simulink model "AFS_DD"  (R2016b)
settings: configuration reference "CodeGenConfigSet" (kept outside this file)
values from neighbouring files (symbols this model uses):
  AFS_facLPFiltPT1_C = Calibration.Parameter    [init_AFS_DD.m]    (also in init_AFS_DD_SIL.m = Simulink.Parameter)
  AFS_tiRawSRCHi_C = Calibration.Parameter    [init_AFS_DD.m]    (also in init_AFS_DD_SIL.m = Simulink.Parameter)
  AFS_tiRawSRCLo_C = Calibration.Parameter    [init_AFS_DD.m]    (also in init_AFS_DD_SIL.m = Simulink.Parameter)
  AFS_tiRawSRCMaxDebDef_C = Calibration.Parameter    [init_AFS_DD.m]    (also in init_AFS_DD_SIL.m = Simulink.Parameter)
  AFS_tiRawSRCMaxDebOk_C = Calibration.Parameter    [init_AFS_DD.m]    (also in init_AFS_DD_SIL.m = Simulink.Parameter)
  AFS_tiRawSRCMinDebDef_C = Calibration.Parameter    [init_AFS_DD.m]    (also in init_AFS_DD_SIL.m = Simulink.Parameter)
  AFS_tiRawSRCMinDebOk_C = Calibration.Parameter    [init_AFS_DD.m]    (also in init_AFS_DD_SIL.m = Simulink.Parameter)
undefined symbols (not defined in the file or in its folder): AFS_DD_DT, Switch_conv
libraries: CXLib x7
settings Model: Creator=Colin  LastModifiedBy=Colin
settings ConfigSetRef: SourceLocation=Base Workspace

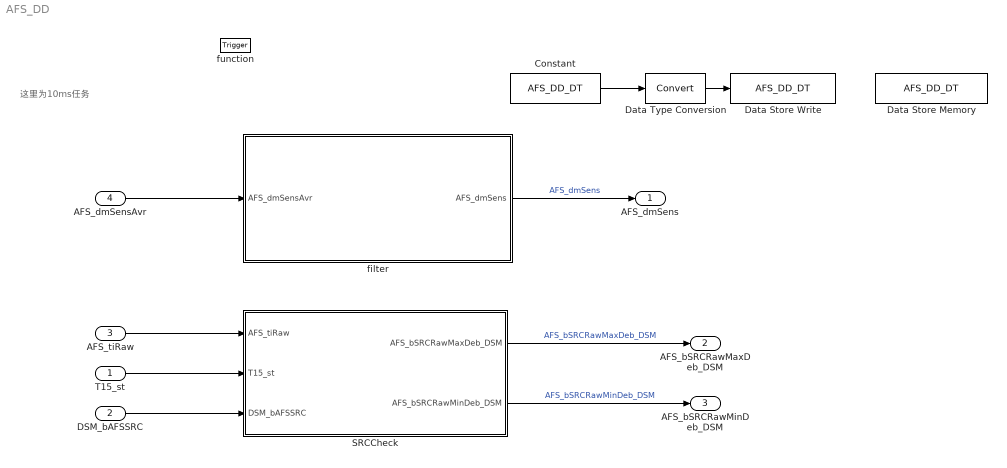
== system AFS_DD ==
  note: 这里为10ms任务
  T15_st : Inport  Description=Terminal 15 status after debouncing  OutDataTypeStr=Enum: Switch_conv
  DSM_bAFSSRC : Inport  Description=Function identifier for inhibition of the signal range check  Port=2  OutMin=0  OutMax=1  OutDataTypeStr=boolean
  AFS_tiRaw : Inport  Tag=us  Description=Raw air mass period  Port=3  OutMin=0  OutMax=107374182  OutDataTypeStr=Time_PwmHigh_us
  AFS_dmSensAvr : Inport  Tag=kg/h  Description=Averaged Sensed air mass flow  Port=4  OutMin=-8192  OutMax=8191  OutDataTypeStr=AirMassPerTime
  function : TriggerPort  TriggerType=function-call  VariantControl=Variant
  Constant : Constant  Value=AFS_DD_DT
  Data Store Memory : DataStoreMemory  DataStoreName=AFS_DD_DT  ReadBeforeWriteMsg=warning  WriteAfterWriteMsg=warning  WriteAfterReadMsg=warning  ShowAdditionalParam=off
  Data Store Write : DataStoreWrite  DataStoreName=AFS_DD_DT
  Data Type Conversion : DataTypeConversion
  SRCCheck : Subsystem
  filter : Subsystem
  AFS_dmSens : Outport  Tag=kg/h  Description=Processed air mass flow signal of the HFM sensor  OutMin=-8192  OutMax=8191  OutDataTypeStr=AirMassPerTime
  AFS_bSRCRawMaxDeb_DSM : Outport  Description=Signal range check high of the air mass flow sensor  Port=2  OutMin=0  OutMax=1  OutDataTypeStr=boolean
  AFS_bSRCRawMinDeb_DSM : Outport  Description=Signal range check low of the air mass flow sensor  Port=3  OutMin=0  OutMax=1  OutDataTypeStr=boolean
  wires:
  T15_st/1 -> SRCCheck/2(T15_st)
  DSM_bAFSSRC/1 -> SRCCheck/3(DSM_bAFSSRC)
  SRCCheck/1(AFS_bSRCRawMaxDeb_DSM) -> AFS_bSRCRawMaxDeb_DSM/1  "AFS_bSRCRawMaxDeb_DSM"
  SRCCheck/2(AFS_bSRCRawMinDeb_DSM) -> AFS_bSRCRawMinDeb_DSM/1  "AFS_bSRCRawMinDeb_DSM"
  Constant/1 -> Data Type Conversion/1
  AFS_tiRaw/1 -> SRCCheck/1(AFS_tiRaw)
  AFS_dmSensAvr/1 -> filter/1(AFS_dmSensAvr)
  filter/1(AFS_dmSens) -> AFS_dmSens/1  "AFS_dmSens"
  Data Type Conversion/1 -> Data Store Write/1

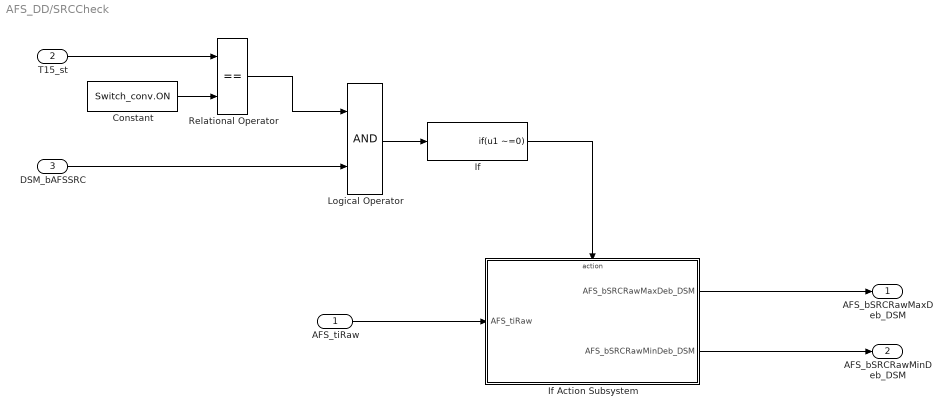
== system AFS_DD/SRCCheck ==
  AFS_tiRaw : Inport
  T15_st : Inport  Port=2
  DSM_bAFSSRC : Inport  Port=3
  Constant : Constant  Value=Switch_conv.ON
  If : If  IfExpression=u1 ~=0  ShowElse=off
  If Action Subsystem : Subsystem  TreatAsAtomicUnit=on
  Logical Operator : Logic  AllPortsSameDT=off  OutDataTypeStr=boolean
  Relational Operator : RelationalOperator  Operator===  OutDataTypeStr=boolean  RndMeth=Simplest
  AFS_bSRCRawMaxDeb_DSM : Outport
  AFS_bSRCRawMinDeb_DSM : Outport  Port=2
  wires:
  T15_st/1 -> Relational Operator/1
  Relational Operator/1 -> Logical Operator/1
  DSM_bAFSSRC/1 -> Logical Operator/2
  Constant/1 -> Relational Operator/2
  AFS_tiRaw/1 -> If Action Subsystem/1(AFS_tiRaw)
  If Action Subsystem/1(AFS_bSRCRawMaxDeb_DSM) -> AFS_bSRCRawMaxDeb_DSM/1
  If Action Subsystem/2(AFS_bSRCRawMinDeb_DSM) -> AFS_bSRCRawMinDeb_DSM/1
  Logical Operator/1 -> If/1
  If/1 -> If Action Subsystem/Action

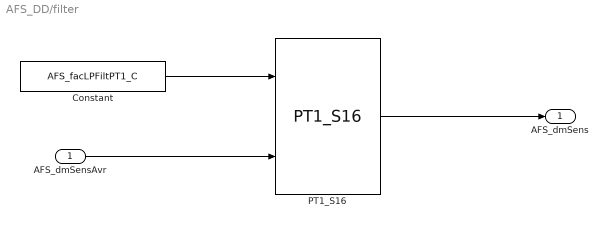
== system AFS_DD/filter ==
  AFS_dmSensAvr : Inport
  Constant : Constant  Value=AFS_facLPFiltPT1_C
  PT1_S16 : CXLib/PT1_S16
  AFS_dmSens : Outport
  wires:
  AFS_dmSensAvr/1 -> PT1_S16/2
  PT1_S16/1 -> AFS_dmSens/1
  Constant/1 -> PT1_S16/1

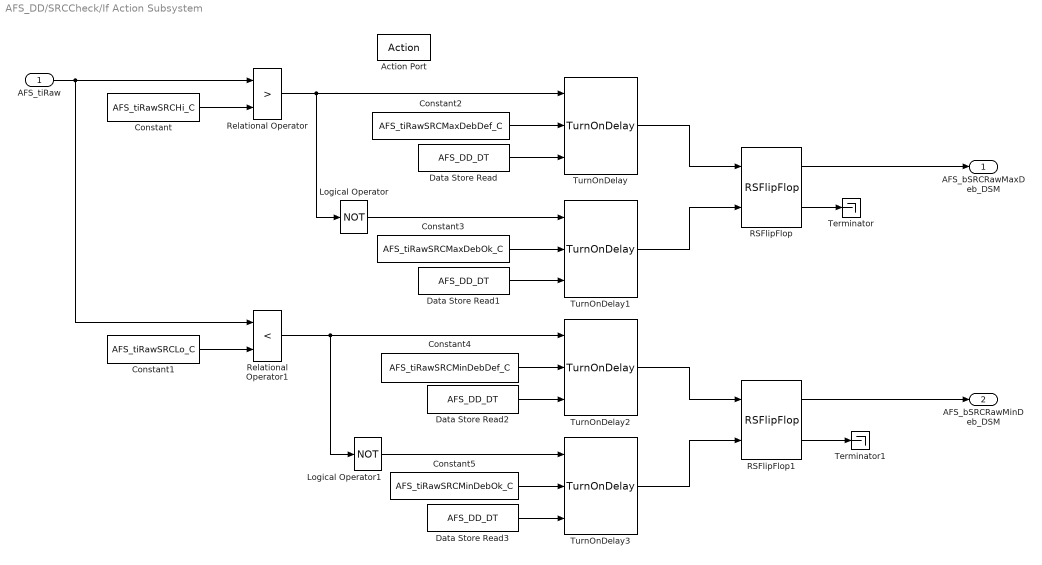
== system AFS_DD/SRCCheck/If Action Subsystem ==
  AFS_tiRaw : Inport
  Action Port : ActionPort  ActionType=then
  Constant : Constant  Value=AFS_tiRawSRCHi_C
  Constant1 : Constant  Value=AFS_tiRawSRCLo_C
  Constant2 : Constant  Value=AFS_tiRawSRCMaxDebDef_C
  Constant3 : Constant  Value=AFS_tiRawSRCMaxDebOk_C
  Constant4 : Constant  Value=AFS_tiRawSRCMinDebDef_C
  Constant5 : Constant  Value=AFS_tiRawSRCMinDebOk_C
  Data Store Read{,1..3} (4 alike) : DataStoreRead  DataStoreName=AFS_DD_DT
  Logical Operator : Logic  Operator=NOT  AllPortsSameDT=off  OutDataTypeStr=boolean
  Logical Operator1 : Logic  Operator=NOT  AllPortsSameDT=off  OutDataTypeStr=boolean
  RSFlipFlop : CXLib/RSFlipFlop
  RSFlipFlop1 : CXLib/RSFlipFlop
  Relational Operator : RelationalOperator  Operator=>  OutDataTypeStr=boolean  RndMeth=Simplest
  Relational Operator1 : RelationalOperator  Operator=<  OutDataTypeStr=boolean  RndMeth=Simplest
  Terminator : Terminator
  Terminator1 : Terminator
  TurnOnDelay{,1..3} (4 alike) : CXLib/TurnOnDelay
  AFS_bSRCRawMaxDeb_DSM : Outport
  AFS_bSRCRawMinDeb_DSM : Outport  Port=2
  wires:
  AFS_tiRaw/1 -> Relational Operator1/1, Relational Operator/1
  Constant/1 -> Relational Operator/2
  Constant1/1 -> Relational Operator1/2
  Constant2/1 -> TurnOnDelay/2
  Data Store Read/1 -> TurnOnDelay/3
  Relational Operator/1 -> Logical Operator/1, TurnOnDelay/1
  Relational Operator1/1 -> Logical Operator1/1, TurnOnDelay2/1
  Logical Operator1/1 -> TurnOnDelay3/1
  Logical Operator/1 -> TurnOnDelay1/1
  Data Store Read1/1 -> TurnOnDelay1/3
  Constant3/1 -> TurnOnDelay1/2
  Constant4/1 -> TurnOnDelay2/2
  Data Store Read2/1 -> TurnOnDelay2/3
  Data Store Read3/1 -> TurnOnDelay3/3
  Constant5/1 -> TurnOnDelay3/2
  TurnOnDelay/1 -> RSFlipFlop/1
  TurnOnDelay1/1 -> RSFlipFlop/2
  RSFlipFlop/2 -> Terminator/1
  RSFlipFlop1/2 -> Terminator1/1
  TurnOnDelay2/1 -> RSFlipFlop1/1
  TurnOnDelay3/1 -> RSFlipFlop1/2
  RSFlipFlop/1 -> AFS_bSRCRawMaxDeb_DSM/1
  RSFlipFlop1/1 -> AFS_bSRCRawMinDeb_DSM/1
